simulink model "simulunk2"  (R2016a)
settings: Solver=VariableStepAuto  StartTime=0.0  StopTime=10.0  RelTol=1e-3
settings Model: Creator=user  LastModifiedBy=user

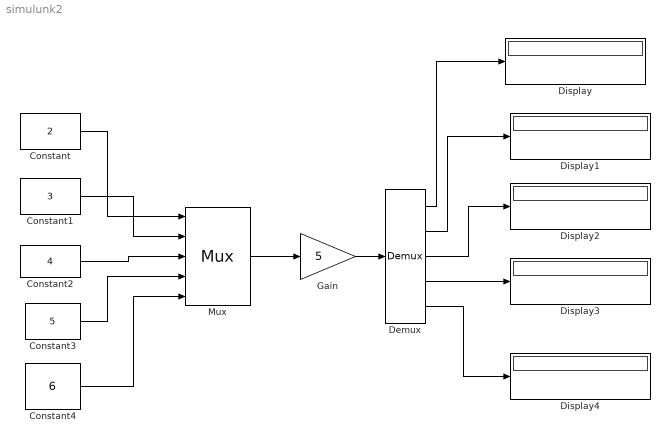
== system simulunk2 ==
  Constant : Constant  Value=2
  Constant1 : Constant  Value=3
  Constant2 : Constant  Value=4
  Constant3 : Constant  Value=5
  Constant4 : Constant  Value=6
  Demux : Demux  Outputs=5
  Display{,1..4} (5 alike) : Display
  Gain : Gain  Gain=5
  Mux : Mux  Inputs=5
  wires:
  Constant4/1 -> Mux/5
  Constant3/1 -> Mux/4
  Constant2/1 -> Mux/3
  Constant1/1 -> Mux/2
  Constant/1 -> Mux/1
  Mux/1 -> Gain/1
  Gain/1 -> Demux/1
  Demux/5 -> Display4/1
  Demux/4 -> Display3/1
  Demux/3 -> Display2/1
  Demux/2 -> Display1/1
  Demux/1 -> Display/1
